simulink model "Adaptive_Controller_Example"  (R2018b)
settings: Solver=FixedStepAuto  StartTime=0.0  StopTime=75  FixedStep=0.01  RelTol=1e-3  EnableMultiTasking=on
PreLoadFcn:
  | R= 2.0; % Ohms
  | L= 0.5; % Henrys
  | Km = .015; % torque constant
  | Kb = .015; % emf constant
  | B = 0.2; % Nms
  | J= 0.02; % kg.m^2
  | Kc= 1;
  | Kf = 0.2;
  | gamma = 0.1;
libraries: simulink x8
settings Model: Creator=cpatel  LastModifiedBy=Trips
settings DataIOCC: LimitDataPoints=on  SaveFormat=Array
settings OptimizationCC: ExpressionDepthLimit=2147483647  LifeSpan=inf
settings DebuggingCC: UnderspecifiedInitializationDetection=Classic  MergeDetectMultiDrivingBlocksExec=none  SolverPrmCheckMsg=warning  StateNameClashWarn=warning  SFUnexpectedBacktrackingDiag=warning  SFNoUnconditionalDefaultTransitionDiag=warning  SFExecutionAtInitializationDiag=none
settings HardwareCC: ProdBitPerPointer=32  ProdBitPerSizeT=32  ProdBitPerPtrDiffT=32  ProdLargestAtomicFloat=None  ProdIntDivRoundTo=Undefined  ProdEndianess=Unspecified  ProdWordSize=32  ProdHWDeviceType=32-bit Generic
settings ModelReferenceCC: PropagateSignalLabelsOutOfModel=off
settings SFSimCC: SimUseLocalCustomCode=off
settings RTWCC: RTWUseLocalCustomCode=off
settings CodeAppCC: StateflowObjectComments=on
settings GRTTargetCC: TargetLangStandard=C89/C90 (ANSI)  GeneratePreprocessorConditionals=Disable all  CombineOutputUpdateFcns=off  GRTInterface=on
settings ConfigComp: CovMetricSettings=dw  CovHtmlReporting=on  CovSaveCumulativeToWorkspaceVar=on  CovSaveSingleToWorkspaceVar=on  CovExternalEMLEnable=off

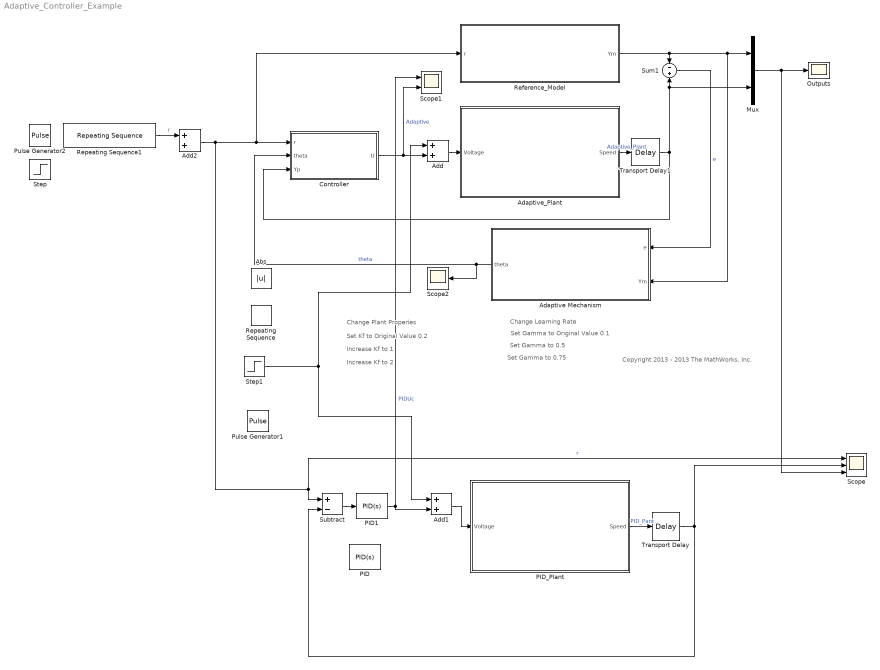
== system Adaptive_Controller_Example ==
  note: Copyright 2013 - 2013 The MathWorks, Inc.
  note: Change Learning Rate
  note: Change Plant Properies
  note: Increase Kf to 1
  note: Set Kf to Original Value 0.2
  note: Increase Kf to 2
  note: Set Gamma to 0.5
  note: Set Gamma to Original Value 0.1
  note: Set Gamma to 0.75
  Abs : Abs
  Adaptive Mechanism : Subsystem
  Adaptive_Plant : Subsystem
  Add : Sum
  Add1 : Sum
  Add2 : Sum
  Controller : Subsystem
  Mux : Mux  Inputs=2
  Outputs : Scope
  PID : simulink/Continuous/PID Controller  Controller=PID  Form=Parallel  TimeDomain=Continuous-time  SampleTime=1  IntegratorMethod=Forward Euler  FilterMethod=Forward Euler  ControllerParametersSource=internal  P=30  I=100  D=0  UseFilter=on  N=100  TunerSelectOption=Transfer Function Based (PID Tuner App)  InitialConditionSource=internal  InitialConditionForIntegrator=0  InitialConditionForFilter=0  DifferentiatorICPrevScaledInput=0  ExternalReset=none  TrackingMode=off  Kt=1  LimitOutput=on  UpperSaturationLimit=600  LowerSaturationLimit=-600  LinearizeAsGain=on  AntiWindupMode=clamping  Kb=1  POutMin=[]  POutMax=[]  IOutMin=[]  IOutMax=[]  DOutMin=[]  DOutMax=[]  NOutMin=[]  NOutMax=[]  SumOutMin=[]  SumOutMax=[]  SaturationOutMin=[]  SaturationOutMax=[]  PParamMin=[]  PParamMax=[]  IParamMin=[]  IParamMax=[]  DParamMin=[]  DParamMax=[]  NParamMin=[]  NParamMax=[]  KbParamMin=[]  KbParamMax=[]  KtParamMin=[]  KtParamMax=[]  KbOutMin=[]  KbOutMax=[]  KtOutMin=[]  KtOutMax=[]  IntegratorOutMin=[]  IntegratorOutMax=[]  FilterOutMin=[]  FilterOutMax=[]  SumI1OutMin=[]  SumI1OutMax=[]  SumI2OutMin=[]  SumI2OutMax=[]  SumI3OutMin=[]  SumI3OutMax=[]  SumI4OutMin=[]  SumI4OutMax=[]  SumDOutMin=[]  SumDOutMax=[]  DifferentiatorOutMin=[]  DifferentiatorOutMax=[]  FilterDiffOutCoefMin=[]  FilterDiffOutCoefMax=[]  ReciprocalOutMin=[]  ReciprocalOutMax=[]  SumDenOutMin=[]  SumDenOutMax=[]  SumNumOutMin=[]  SumNumOutMax=[]  DivideOutMin=[]  DivideOutMax=[]  IntegratorContinuousStateAttributes=''  IntegratorStateMustResolveToSignalObject=off  IntegratorRTWStateStorageClass=Auto  FilterContinuousStateAttributes=''  FilterStateMustResolveToSignalObject=off  FilterRTWStateStorageClass=Auto  ParallelPVariant=InternalParameters  IdealPVariant=Disabled  IVariant=InternalParameters  DVariant=InternalParameters  IntegratorVariant=Continuous  SatVariant=Enabled  AWVariant=ContClampingParallel  PCopyVariant=Disabled  TRVariant=Disabled  FdbkBlocksVariant=Forward  IdealPFdbkVariant=Disabled  SatFdbkVariant=Disabled  DerivativeFilterVariant=ContFilter  NVariant=InternalParameters  NCopyVariant=Disabled  FilterICVariant=InternalICsFilter  IntegratorICVariant=InternalICs  ExternalResetVariant=Disabled  TRSumVariant=Passthrough  SumFdbkVariant=Disabled  SumVariant=Sum_PID
  PID1 : simulink/Continuous/PID Controller  Controller=PID  Form=Parallel  TimeDomain=Continuous-time  SampleTime=1  IntegratorMethod=Forward Euler  FilterMethod=Forward Euler  ControllerParametersSource=internal  P=11.3892413451779  I=15.7050092150697  D=-4.79192148497946  UseFilter=on  N=0.663164279868992  TunerSelectOption=Transfer Function Based (PID Tuner App)  InitialConditionSource=internal  InitialConditionForIntegrator=0  InitialConditionForFilter=0  DifferentiatorICPrevScaledInput=0  ExternalReset=none  TrackingMode=off  Kt=1  LimitOutput=on  UpperSaturationLimit=600  LowerSaturationLimit=-600  LinearizeAsGain=on  AntiWindupMode=clamping  Kb=1  POutMin=[]  POutMax=[]  IOutMin=[]  IOutMax=[]  DOutMin=[]  DOutMax=[]  NOutMin=[]  NOutMax=[]  SumOutMin=[]  SumOutMax=[]  SaturationOutMin=[]  SaturationOutMax=[]  PParamMin=[]  PParamMax=[]  IParamMin=[]  IParamMax=[]  DParamMin=[]  DParamMax=[]  NParamMin=[]  NParamMax=[]  KbParamMin=[]  KbParamMax=[]  KtParamMin=[]  KtParamMax=[]  KbOutMin=[]  KbOutMax=[]  KtOutMin=[]  KtOutMax=[]  IntegratorOutMin=[]  IntegratorOutMax=[]  FilterOutMin=[]  FilterOutMax=[]  SumI1OutMin=[]  SumI1OutMax=[]  SumI2OutMin=[]  SumI2OutMax=[]  SumI3OutMin=[]  SumI3OutMax=[]  SumI4OutMin=[]  SumI4OutMax=[]  SumDOutMin=[]  SumDOutMax=[]  DifferentiatorOutMin=[]  DifferentiatorOutMax=[]  FilterDiffOutCoefMin=[]  FilterDiffOutCoefMax=[]  ReciprocalOutMin=[]  ReciprocalOutMax=[]  SumDenOutMin=[]  SumDenOutMax=[]  SumNumOutMin=[]  SumNumOutMax=[]  DivideOutMin=[]  DivideOutMax=[]  IntegratorContinuousStateAttributes=''  IntegratorStateMustResolveToSignalObject=off  IntegratorRTWStateStorageClass=Auto  FilterContinuousStateAttributes=''  FilterStateMustResolveToSignalObject=off  FilterRTWStateStorageClass=Auto  ParallelPVariant=InternalParameters  IdealPVariant=Disabled  IVariant=InternalParameters  DVariant=InternalParameters  IntegratorVariant=Continuous  SatVariant=Enabled  AWVariant=ContClampingParallel  PCopyVariant=Disabled  TRVariant=Disabled  FdbkBlocksVariant=Forward  IdealPFdbkVariant=Disabled  SatFdbkVariant=Disabled  DerivativeFilterVariant=ContFilter  NVariant=InternalParameters  NCopyVariant=Disabled  FilterICVariant=InternalICsFilter  IntegratorICVariant=InternalICs  ExternalResetVariant=Disabled  TRSumVariant=Passthrough  SumFdbkVariant=Disabled  SumVariant=Sum_PID
  PID_Plant : Subsystem
  Pulse Generator1 : DiscretePulseGenerator  PulseType=Time based  Amplitude=3  Period=5  PulseWidth=50
  Pulse Generator2 : DiscretePulseGenerator  PulseType=Time based  Amplitude=3.14  Period=10  PulseWidth=50
  Reference_Model : Subsystem
  Repeating Sequence : simulink/Sources/Repeating Sequence  rep_seq_t=[ 0 15 25 75]  rep_seq_y=[0 0 50 0 ]
  Repeating Sequence1 : simulink/Sources/Repeating Sequence  rep_seq_t=[0 19 20 29 30 39 40 49 50 60]  rep_seq_y="[3  3  4  4   3   3   2  2  3 3]"
  Scope : Scope  NumInputPorts=3
  Scope1 : Scope  NumInputPorts=2
  Scope2 : Scope
  Step : Step  Time=0  After=3.14  SampleTime=0
  Step1 : Step  Time=15  After=30  SampleTime=0
  Subtract : Sum  Inputs=+-
  Sum1 : Sum  Inputs=-|+
  Transport Delay : TransportDelay
  Transport Delay1 : TransportDelay
  wires:
  Mux/1 -> Scope/3, Outputs/1
  Adaptive Mechanism/1(theta) -> Controller/2(theta), Scope2/1  "theta"
  Sum1/1 -> Adaptive Mechanism/1(e)  "e"
  Controller/1(U) -> Scope1/2, Add/2  "Adaptive"
  Add/1 -> Adaptive_Plant/1(Voltage)
  PID1/1 -> Add1/2, Scope1/1  "PIDUc"
  Subtract/1 -> PID1/1
  Add2/1 -> Subtract/1, Scope/1, Reference_Model/1(r), Controller/1(r)  "r"
  PID_Plant/1(Speed) -> Transport Delay/1  "PID_Pant"
  Step1/1 -> Add1/1, Add/1
  Add1/1 -> PID_Plant/1(Voltage)
  Repeating Sequence1/1 -> Add2/1  "r"
  Adaptive_Plant/1(Speed) -> Transport Delay1/1  "Adaptive_Plant"
  Reference_Model/1(Ym) -> Sum1/1, Adaptive Mechanism/2(Ym), Mux/1
  Transport Delay/1 -> Scope/2, Subtract/2
  Transport Delay1/1 -> Sum1/2, Mux/2, Controller/3(Yp)

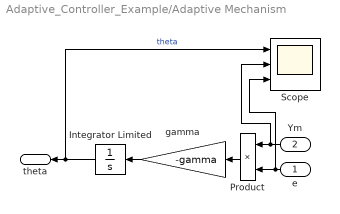
== system Adaptive_Controller_Example/Adaptive Mechanism ==
  e : Inport
  Ym : Inport  Port=2
  Integrator Limited : Integrator  LimitOutput=on  UpperSaturationLimit=100  LowerSaturationLimit=-100
  Product : Product
  Scope : Scope  NumInputPorts=3
  gamma : Gain  Gain=-gamma
  theta : Outport
  wires:
  Integrator Limited/1 -> Scope/1, theta/1  "theta"
  gamma/1 -> Integrator Limited/1
  Product/1 -> gamma/1
  Ym/1 -> Scope/2, Product/1
  e/1 -> Scope/3, Product/2

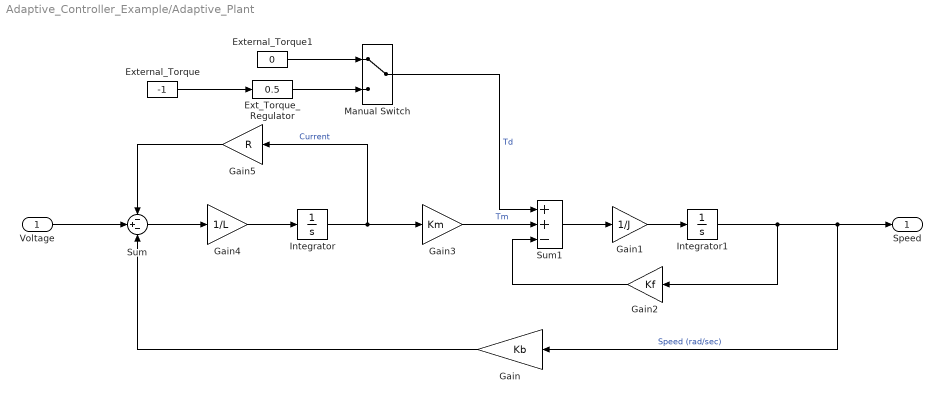
== system Adaptive_Controller_Example/Adaptive_Plant ==
  Voltage : Inport
  Ext_Torque_Regulator : simulink/Math Operations/Slider Gain  gain=0.5  low=0  high=1
  External_Torque : Constant  Value=-1
  External_Torque1 : Constant  Value=0
  Gain : Gain  Gain=Kb
  Gain1 : Gain  Gain=1/J
  Gain2 : Gain  Gain=Kf
  Gain3 : Gain  Gain=Km
  Gain4 : Gain  Gain=1/L
  Gain5 : Gain  Gain=R
  Integrator : Integrator  ContinuousStateAttributes='Current'
  Integrator1 : Integrator  ContinuousStateAttributes='Speed'
  Manual Switch : ManualSwitch
  Sum : Sum  Inputs=-+-
  Sum1 : Sum  Inputs=++-
  Speed : Outport
  wires:
  Sum/1 -> Gain4/1
  Gain3/1 -> Sum1/2  "Tm"
  Sum1/1 -> Gain1/1
  Integrator1/1 -> Gain/1, Speed/1, Gain2/1  "Speed (rad/sec)"
  Gain1/1 -> Integrator1/1
  Gain2/1 -> Sum1/3
  Integrator/1 -> Gain3/1, Gain5/1  "Current"
  Gain4/1 -> Integrator/1
  Gain/1 -> Sum/3
  Voltage/1 -> Sum/2
  Gain5/1 -> Sum/1
  Manual Switch/1 -> Sum1/1  "Td"
  External_Torque/1 -> Ext_Torque_Regulator/1
  External_Torque1/1 -> Manual Switch/1
  Ext_Torque_Regulator/1 -> Manual Switch/2

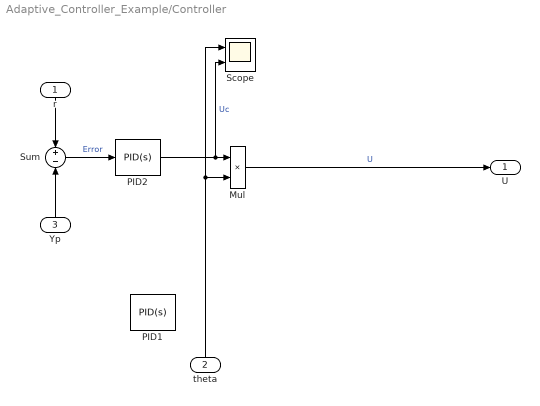
== system Adaptive_Controller_Example/Controller ==
  r : Inport
  theta : Inport  Port=2
  Yp : Inport  Port=3
  Mul : Product
  PID1 : simulink/Continuous/PID Controller  Controller=PID  Form=Parallel  TimeDomain=Continuous-time  SampleTime=1  IntegratorMethod=Forward Euler  FilterMethod=Forward Euler  ControllerParametersSource=internal  P=30  I=100  D=0  UseFilter=on  N=100  TunerSelectOption=Transfer Function Based (PID Tuner App)  InitialConditionSource=internal  InitialConditionForIntegrator=0  InitialConditionForFilter=0  DifferentiatorICPrevScaledInput=0  ExternalReset=none  TrackingMode=off  Kt=1  LimitOutput=on  UpperSaturationLimit=600  LowerSaturationLimit=-600  LinearizeAsGain=on  AntiWindupMode=clamping  Kb=1  POutMin=[]  POutMax=[]  IOutMin=[]  IOutMax=[]  DOutMin=[]  DOutMax=[]  NOutMin=[]  NOutMax=[]  SumOutMin=[]  SumOutMax=[]  SaturationOutMin=[]  SaturationOutMax=[]  PParamMin=[]  PParamMax=[]  IParamMin=[]  IParamMax=[]  DParamMin=[]  DParamMax=[]  NParamMin=[]  NParamMax=[]  KbParamMin=[]  KbParamMax=[]  KtParamMin=[]  KtParamMax=[]  KbOutMin=[]  KbOutMax=[]  KtOutMin=[]  KtOutMax=[]  IntegratorOutMin=[]  IntegratorOutMax=[]  FilterOutMin=[]  FilterOutMax=[]  SumI1OutMin=[]  SumI1OutMax=[]  SumI2OutMin=[]  SumI2OutMax=[]  SumI3OutMin=[]  SumI3OutMax=[]  SumI4OutMin=[]  SumI4OutMax=[]  SumDOutMin=[]  SumDOutMax=[]  DifferentiatorOutMin=[]  DifferentiatorOutMax=[]  FilterDiffOutCoefMin=[]  FilterDiffOutCoefMax=[]  ReciprocalOutMin=[]  ReciprocalOutMax=[]  SumDenOutMin=[]  SumDenOutMax=[]  SumNumOutMin=[]  SumNumOutMax=[]  DivideOutMin=[]  DivideOutMax=[]  IntegratorContinuousStateAttributes=''  IntegratorStateMustResolveToSignalObject=off  IntegratorRTWStateStorageClass=Auto  FilterContinuousStateAttributes=''  FilterStateMustResolveToSignalObject=off  FilterRTWStateStorageClass=Auto  ParallelPVariant=InternalParameters  IdealPVariant=Disabled  IVariant=InternalParameters  DVariant=InternalParameters  IntegratorVariant=Continuous  SatVariant=Enabled  AWVariant=ContClampingParallel  PCopyVariant=Disabled  TRVariant=Disabled  FdbkBlocksVariant=Forward  IdealPFdbkVariant=Disabled  SatFdbkVariant=Disabled  DerivativeFilterVariant=ContFilter  NVariant=InternalParameters  NCopyVariant=Disabled  FilterICVariant=InternalICsFilter  IntegratorICVariant=InternalICs  ExternalResetVariant=Disabled  TRSumVariant=Passthrough  SumFdbkVariant=Disabled  SumVariant=Sum_PID
  PID2 : simulink/Continuous/PID Controller  Controller=PID  Form=Parallel  TimeDomain=Continuous-time  SampleTime=1  IntegratorMethod=Forward Euler  FilterMethod=Forward Euler  ControllerParametersSource=internal  P=11.3892413451779  I=15.7050092150697  D=-4.79192148497946  UseFilter=on  N=0.663164279868992  TunerSelectOption=Transfer Function Based (PID Tuner App)  InitialConditionSource=internal  InitialConditionForIntegrator=0  InitialConditionForFilter=0  DifferentiatorICPrevScaledInput=0  ExternalReset=none  TrackingMode=off  Kt=1  LimitOutput=on  UpperSaturationLimit=600  LowerSaturationLimit=-600  LinearizeAsGain=on  AntiWindupMode=clamping  Kb=1  POutMin=[]  POutMax=[]  IOutMin=[]  IOutMax=[]  DOutMin=[]  DOutMax=[]  NOutMin=[]  NOutMax=[]  SumOutMin=[]  SumOutMax=[]  SaturationOutMin=[]  SaturationOutMax=[]  PParamMin=[]  PParamMax=[]  IParamMin=[]  IParamMax=[]  DParamMin=[]  DParamMax=[]  NParamMin=[]  NParamMax=[]  KbParamMin=[]  KbParamMax=[]  KtParamMin=[]  KtParamMax=[]  KbOutMin=[]  KbOutMax=[]  KtOutMin=[]  KtOutMax=[]  IntegratorOutMin=[]  IntegratorOutMax=[]  FilterOutMin=[]  FilterOutMax=[]  SumI1OutMin=[]  SumI1OutMax=[]  SumI2OutMin=[]  SumI2OutMax=[]  SumI3OutMin=[]  SumI3OutMax=[]  SumI4OutMin=[]  SumI4OutMax=[]  SumDOutMin=[]  SumDOutMax=[]  DifferentiatorOutMin=[]  DifferentiatorOutMax=[]  FilterDiffOutCoefMin=[]  FilterDiffOutCoefMax=[]  ReciprocalOutMin=[]  ReciprocalOutMax=[]  SumDenOutMin=[]  SumDenOutMax=[]  SumNumOutMin=[]  SumNumOutMax=[]  DivideOutMin=[]  DivideOutMax=[]  IntegratorContinuousStateAttributes=''  IntegratorStateMustResolveToSignalObject=off  IntegratorRTWStateStorageClass=Auto  FilterContinuousStateAttributes=''  FilterStateMustResolveToSignalObject=off  FilterRTWStateStorageClass=Auto  ParallelPVariant=InternalParameters  IdealPVariant=Disabled  IVariant=InternalParameters  DVariant=InternalParameters  IntegratorVariant=Continuous  SatVariant=Enabled  AWVariant=ContClampingParallel  PCopyVariant=Disabled  TRVariant=Disabled  FdbkBlocksVariant=Forward  IdealPFdbkVariant=Disabled  SatFdbkVariant=Disabled  DerivativeFilterVariant=ContFilter  NVariant=InternalParameters  NCopyVariant=Disabled  FilterICVariant=InternalICsFilter  IntegratorICVariant=InternalICs  ExternalResetVariant=Disabled  TRSumVariant=Passthrough  SumFdbkVariant=Disabled  SumVariant=Sum_PID
  Scope : Scope  NumInputPorts=2
  Sum : Sum  Inputs=+|-
  U : Outport
  wires:
  theta/1 -> Scope/1, Mul/2
  r/1 -> Sum/1
  Yp/1 -> Sum/2
  Sum/1 -> PID2/1  "Error"
  Mul/1 -> U/1  "U"
  PID2/1 -> Scope/2, Mul/1  "Uc"

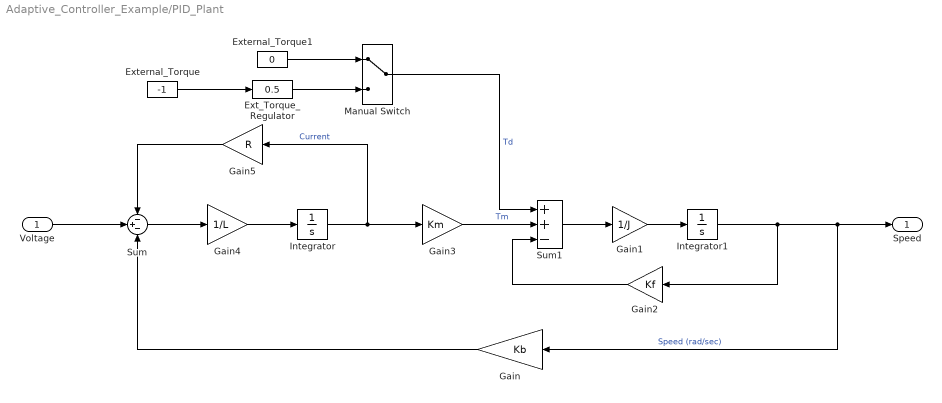
== system Adaptive_Controller_Example/PID_Plant ==
  Voltage : Inport
  Ext_Torque_Regulator : simulink/Math Operations/Slider Gain  gain=0.5  low=0  high=1
  External_Torque : Constant  Value=-1
  External_Torque1 : Constant  Value=0
  Gain : Gain  Gain=Kb
  Gain1 : Gain  Gain=1/J
  Gain2 : Gain  Gain=Kf
  Gain3 : Gain  Gain=Km
  Gain4 : Gain  Gain=1/L
  Gain5 : Gain  Gain=R
  Integrator : Integrator  ContinuousStateAttributes='Current'
  Integrator1 : Integrator  ContinuousStateAttributes='Speed'
  Manual Switch : ManualSwitch
  Sum : Sum  Inputs=-+-
  Sum1 : Sum  Inputs=++-
  Speed : Outport
  wires:
  Sum/1 -> Gain4/1
  Gain3/1 -> Sum1/2  "Tm"
  Sum1/1 -> Gain1/1
  Integrator1/1 -> Gain/1, Speed/1, Gain2/1  "Speed (rad/sec)"
  Gain1/1 -> Integrator1/1
  Gain2/1 -> Sum1/3
  Integrator/1 -> Gain3/1, Gain5/1  "Current"
  Gain4/1 -> Integrator/1
  Gain/1 -> Sum/3
  Voltage/1 -> Sum/2
  Gain5/1 -> Sum/1
  Manual Switch/1 -> Sum1/1  "Td"
  External_Torque/1 -> Ext_Torque_Regulator/1
  External_Torque1/1 -> Manual Switch/1
  Ext_Torque_Regulator/1 -> Manual Switch/2

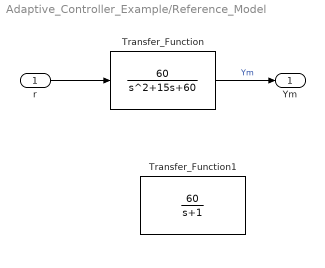
== system Adaptive_Controller_Example/Reference_Model ==
  r : Inport
  Transfer_Function : TransferFcn  Numerator=[60]  Denominator=[1 15 60]
  Transfer_Function1 : TransferFcn  Numerator=[60]  Denominator=[1 1]
  Ym : Outport
  wires:
  Transfer_Function/1 -> Ym/1  "Ym"
  r/1 -> Transfer_Function/1
